simulink model "temp8"  (Simulink 7.7)
settings: Solver=ode45  SolverMode=SingleTasking  StartTime=0.0  StopTime=50  RelTol=1e-3
PreLoadFcn:
  | RefSignals
model workspace (MATLAB code in the model file):
  | commdvbt_tablegen
values from neighbouring files (symbols this model uses):
  Tsample = 9e3    (= 9000)    [RefSignals.m]
  VAR = {}    [RefSignals.m]
undefined symbols (not defined in the file or in its folder): Fs, get, rsgenpoly, sided, Two
libraries: dspmtrx3 x16, simulink x9, commblkintrlv2 x3, commutil2 x3, commblkcod2 x1, commcnvcod2 x1, commdigbbndam3 x1, dspxfrm3 x1, dspsnks4 x1, dspsigops x1, commcnvintrlv2 x1, commsdrhw_v2 x1
Description:
  | Digital Video Broadcasting - Terrestrial
CloseFcn:
  | % Clear global variables
  | clear global GF_TABLE1 GF_TABLE2 GF_TABLE_M GF_TABLE_PRIM_POLY
  | 
  | % Clear signal logging variable
  | clear dvbSigsOut
settings Model: Creator=The MathWorks Inc.  LastModifiedBy=katsikas  ExtModeTrigMode=oneshot  ExtModeArmWhenConnect=off  ExtModeAutoUpdateStatusClock=off  BufferReuse=off
settings SolverCC: ZeroCrossControl=DisableAll
settings DataIOCC: LimitDataPoints=off  SaveOutput=off  SaveTime=off  SignalLoggingName=dvbSigsOut
settings OptimizationCC: BlockReduction=off  BooleanDataType=off  OptimizeBlockIOStorage=off  BufferReuse=off  ExpressionFolding=off  LocalBlockOutputs=off  InitFltsAndDblsToZero=on  EfficientMapNaN2IntZero=off  OptimizeModelRefInitCode=on  LifeSpan=1  BufferReusableBoundary=off
settings DebuggingCC: SaveWithParameterizedLinksMsg=none  CheckExecutionContextPreStartOutputMsg=on  CheckExecutionContextRuntimeOutputMsg=on  SignalResolutionControl=TryResolveAllWithWarning  SolverPrmCheckMsg=none  InheritedTsInSrcMsg=none  MultiTaskDSMMsg=warning  MultiTaskCondExecSysMsg=none  SigSpecEnsureSampleTimeMsg=none  BusObjectLabelMismatch=none  StrictBusMsg=None
settings HardwareCC: TargetBitPerLong=64  TargetBitPerPointer=64  TargetEndianess=LittleEndian  TargetWordSize=64  TargetHWDeviceType=MATLAB Host
settings ModelReferenceCC: UpdateModelReferenceTargets=IfOutOfDate
settings RTWCC: SystemTargetFile=ert.tlc  TemplateMakefile=ert_default_tmf  Description=Real-Time Workshop Embedded Coder (no auto configuration)  RetainRTWFile=on  ProcessScript=ert_make_rtw_hook  IncludeERTFirstTime=on
settings CodeAppCC: IgnoreCustomStorageClasses=off
settings ERTTargetCC: TargetFcnLib=ansi_tfl_tmw.mat  FunctionExecutionProfile=off  MultiwordLength=2048  GenerateSampleERTMain=on  MatFileLogging=on  InlinedParameterPlacement=NonHierarchical  ERTCustomFileTemplate=example_file_process.tlc  ConvertIfToSwitch=off

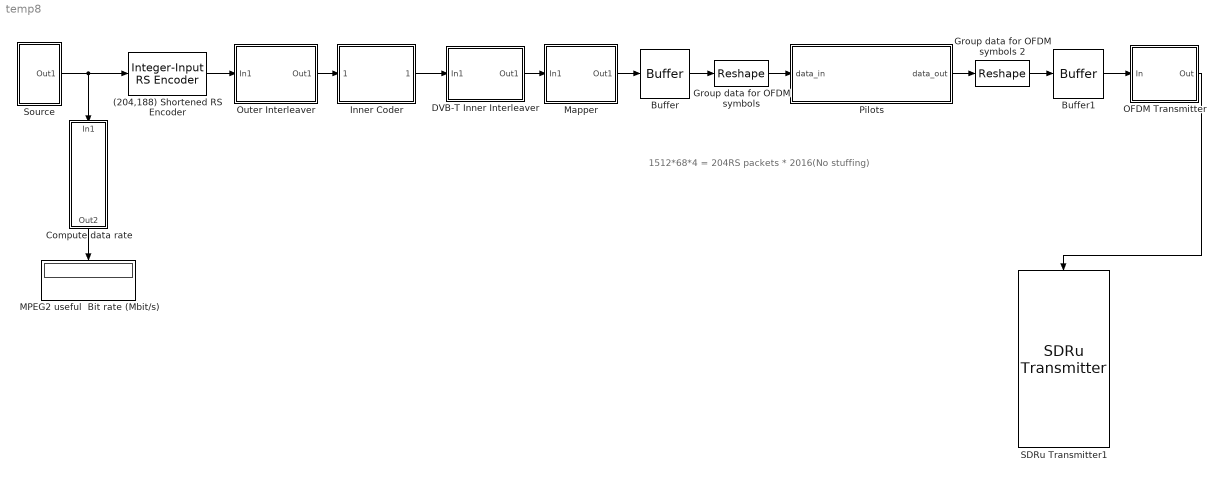
== system temp8 ==
  note: 1512*68*4 = 204RS packets * 2016(No stuffing)
  (204,188) Shortened RS Encoder : commblkcod2/Integer-Input RS Encoder  n=204  k=188  specPrimPoly=off  prPoly=[1 0 1 1]  specGenPoly=off  genPoly=rsgenpoly(7,3)  specPuncture=off  punctVec=[ones(2,1); zeros(2,1)]
  Buffer : Buffer  N=1512*68  TreatMby1Signals=One channel
  Buffer1 : Buffer  N=1705  TreatMby1Signals=One channel
  Compute data rate : Subsystem
      mask Display: disp(sprintf('Compute Bit\nRate (Mbit/s)'))
  DVB-T Inner Interleaver : Subsystem  mask(DVB-T Inner Interleaver){}
      mask init:
      | fullILVec = [(1:126) ...
      |  (rem([0:125]+63,126) +1 + 126     ) ...
      |  (rem([0:125]+105,126)+1 + (2*126) ) ...
      |  (rem([0:125]+42,126) +1 + (3*126) ) ...
      |  (rem([0:125]+21,126) +1 + (4*126) ) ...
      |  (rem([0:125]+84,126) +1 + (5*126) )];
      mask Display: disp('DVB-T\nInner\nInterleaver')
  "Group data for OFDM symbols " : Reshape  OutputDimensionality=Customize  OutputDimensions=[1512 68]
  Group data for OFDM symbols 2 : Reshape  OutputDimensionality=Column vector (2-D)  OutputDimensions=[1512 68]
  Inner Coder : Subsystem
      mask Display: disp('Rate 3/4\nPunctured\nConvolutional\nCode');
  MPEG2 useful  Bit rate (Mbit/s) : Display
      settings: Format=bank
  Mapper : Subsystem
      mask Type: DVB-T 64-QAM Mapper
      mask Display: disp('DVB-T\n64-QAM\nMapper')
  OFDM Transmitter : Subsystem
      mask Display: disp('OFDM\nTransmitter')
  Outer Interleaver : Subsystem
      mask Display: disp('Convolutional\nInterleaver\nI=12')
  Pilots : Stateflow chart  TreatAsAtomicUnit=on
  SDRu Transmitter1 : commsdrhw_v2/SDRu Transmitter  SystemSampleTime=-1  rxtx=tx  USRP2_IP='192.168.10.2'  centerFrequency=474e6  centerFrequencySrc=Dialog  loOffset=0  loOffsetSrc=Dialog  gain=20  gainSrc=Dialog  decimInterp=512  decimInterpSrc=Dialog  USRP2_IP_NUM=[49 57 50 46 49 54 56 46 49 48 46 50]  frameLength=362  outputDatatype=int16  overrunUnderrunPort=off  sampleTime=1  dboardInfo=|  HOST_DATA_PORT=30000  HOST_CONTROL_PORT=30001  USRP2_DATA_PORT=32769  USRP2_CONTROL_PORT=32768
      | dbid: 0
      |           dbName: 'no db found'
      |          freqMin: 0
      |          freqMax: 0
      |          gainMin: 0
      |          gainMax: 0
      |     gainStepSize: 0
  Source : Subsystem
  wires:
  Source/1(Out1) -> Compute data rate/1(In1), (204,188) Shortened RS Encoder/1
  (204,188) Shortened RS Encoder/1 -> Outer Interleaver/1(In1)
  Outer Interleaver/1(Out1) -> Inner Coder/1(Uncoded symbols)
  ? -> ?
  DVB-T Inner Interleaver/1(Out1) -> Mapper/1(In1)
  Inner Coder/1(Coded bits) -> DVB-T Inner Interleaver/1(In1)
  Mapper/1(Out1) -> Buffer/1
  Buffer/1 -> "Group data for OFDM symbols "/1
  "Group data for OFDM symbols "/1 -> Pilots/1(data_in)
  Pilots/1(data_out) -> Group data for OFDM symbols 2/1
  Compute data rate/1(Out2) -> MPEG2 useful  Bit rate (Mbit/s)/1
  OFDM Transmitter/1(Out) -> SDRu Transmitter1/1
  Buffer1/1 -> OFDM Transmitter/1(In)
  Group data for OFDM symbols 2/1 -> Buffer1/1

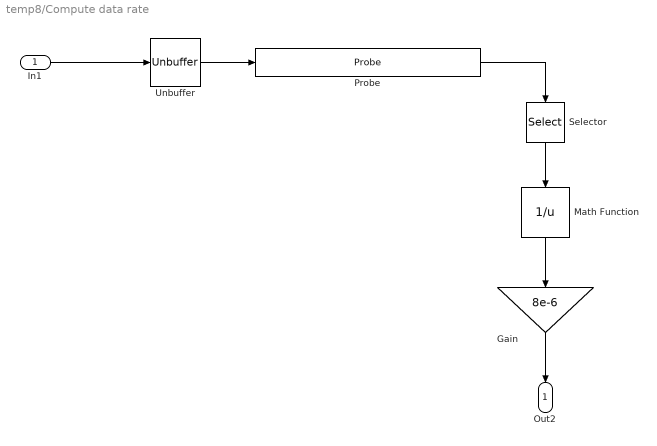
== system temp8/Compute data rate ==
  In1 : Inport
  Gain : Gain  Gain=8e-6
  Math Function : Math  Operator=reciprocal  SaturateOnIntegerOverflow=on
  Probe : Probe  ProbeWidth=off  ProbeComplexSignal=off
  Selector : Selector  InputPortWidth=2  IndexOptions=Index vector (dialog)  Indices=1  OutputSizes=1
  Unbuffer : Unbuffer  SampleBasedProcessing=Same as frame based
  Out2 : Outport
  wires:
  Probe/1 -> Selector/1
  In1/1 -> Unbuffer/1
  Selector/1 -> Math Function/1
  Math Function/1 -> Gain/1
  Gain/1 -> Out2/1
  Unbuffer/1 -> Probe/1

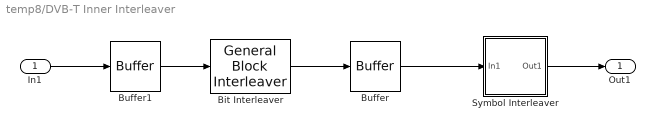
== system temp8/DVB-T Inner Interleaver ==
  In1 : Inport
  Bit Interleaver : commblkintrlv2/General Block Interleaver  elements=dvb_bit_int_table
  Buffer : Buffer  N=9072  TreatMby1Signals=One channel
  Buffer1 : Buffer  N=756  TreatMby1Signals=One channel
  Symbol Interleaver : Subsystem
      mask Display:
      | port_label('input', 1, '')
      | port_label('output', 1, '')
      | disp('Symbol\nInterleaver')
  Out1 : Outport
  wires:
  Buffer1/1 -> Bit Interleaver/1
  In1/1 -> Buffer1/1
  Bit Interleaver/1 -> Buffer/1
  Symbol Interleaver/1(Out1) -> Out1/1
  Buffer/1 -> Symbol Interleaver/1(In1)

== system temp8/Inner Coder ==
  Uncoded symbols : Inport
  Convolutional  Encoder : commcnvcod2/Convolutional Encoder  trellis=poly2trellis(7, [171 133])  opMode=Continuous  DelayedResetAction=off  hasIniStPort=off  hasFinStPort=off  usePuncVector=on  punctureVector=[1 1 0 1 1 0]'  reset=Unused parameter value
  Coded bits : Outport
  wires:
  Convolutional  Encoder/1 -> Coded bits/1
  Uncoded symbols/1 -> Convolutional  Encoder/1

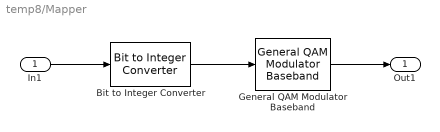
== system temp8/Mapper ==
  In1 : Inport
  Bit to Integer Converter : commutil2/Bit to Integer Converter  nbits=6  bitOrder=MSB first  signedOutputValues=Unsigned  outDtype=uint8  outDtypeSigned=Inherit via internal rule
  General QAM Modulator Baseband : commdigbbndam3/General QAM Modulator Baseband  SigCon=dvbt_qam  outDtype=double  outWordLen=16  outUDDataType=sfix(16)  outFracLenMode=Best precision  outFracLen=15
  Out1 : Outport
  wires:
  General QAM Modulator Baseband/1 -> Out1/1
  In1/1 -> Bit to Integer Converter/1
  Bit to Integer Converter/1 -> General QAM Modulator Baseband/1

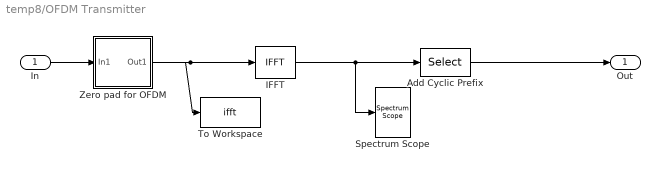
== system temp8/OFDM Transmitter ==
  In : Inport
  Add Cyclic Prefix : Selector  NumberOfDimensions=2  InputPortWidth=64  IndexOptions=Index vector (dialog),Select all  Indices=VAR.CyclicPrefixTX,-1  OutputSizes=1
  IFFT : dspxfrm3/IFFT  CompMethod=Table lookup  TableOpt=HYBRID  TableOptActive=Speed  BitRevOrder=off  cs_in=off  SkipNorm=on  InheritFFTLength=on  FFTLength=64  mode=Complex  outSamplingMode=Frame based  RowConvenienceOn=on  firstCoeffMode=User-defined  firstCoeffWordLength=16  firstCoeffFracLength=15  firstCoeffDataTypeStr=fixdt(1,16)  firstCoeffLastDataTypeStr=fixdt(1,16)  outputMin=[]  outputMax=[]  accumDataTypeStr=Inherit: Same as product output  accumLastDataTypeStr=Inherit: Same as product output  roundingMode=Floor  overflowMode=off
  Spectrum Scope : dspsnks4/Spectrum Scope  SystemSampleTime=-1  ScopeProperties=on  Domain=Frequency  HorizSpan=1  UseBuffer=off  BufferSize=128  Overlap=0  TreatMby1Signals=One channel  inpFftLenInherit=off  FFTlength=128  numAvg=2  DisplayProperties=off  AxisGrid=on  Memory=off  FrameNumber=on  AxisLegend=off  AxisZoom=off  OpenScopeAtSimStart=on  OpenScopeImmediately=off  FigPos=get(0,'defaultfigureposition')  AxisProperties=off  XUnits=Hertz  XRange=Two-sided ((-Fs/2...Fs/2])  XDisplay=0  InheritXIncr=on  XIncr=1.0  XLabel=Samples  XLimit=Auto  YUnits=dBW/Hertz  XMax=1  XMin=0  YLabel=Magnitude-squared, dB  LineProperties=off  wintypeSpecScope=Hann  RsSpecScope=50  betaSpecScope=5  winsampSpecScope=Periodic  XAxisParamsVer=6.9  isFrameUpgraded=on
      settings: YMin=-10  YMax=10
  To Workspace : ToWorkspace  VariableName=ifft  SampleTime=-1  SaveFormat=Array
  Zero pad for OFDM : Subsystem
      mask Display: disp('Zero pad\nfor OFDM');
  Out : Outport
  wires:
  IFFT/1 -> Add Cyclic Prefix/1, Spectrum Scope/1
  In/1 -> Zero pad for OFDM/1(In1)
  Zero pad for OFDM/1(Out1) -> IFFT/1, To Workspace/1
  Add Cyclic Prefix/1 -> Out/1

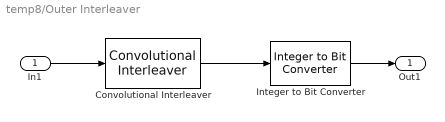
== system temp8/Outer Interleaver ==
  In1 : Inport
  Convolutional Interleaver : commcnvintrlv2/Convolutional Interleaver  SystemSampleTime=-1  N=12  B=17  ic=0
  Integer to Bit Converter : commutil2/Integer to Bit Converter  nbits=8  signedInputValues=Unsigned  bitOrder=MSB first  outDtype=boolean
  Out1 : Outport
  wires:
  Integer to Bit Converter/1 -> Out1/1
  Convolutional Interleaver/1 -> Integer to Bit Converter/1
  In1/1 -> Convolutional Interleaver/1

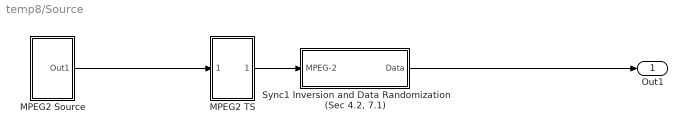
== system temp8/Source ==
  MPEG2 Source : Subsystem
  MPEG2 TS : Subsystem
  "Sync1 Inversion and Data Randomization (Sec 4.2, 7.1)" : Subsystem
  Out1 : Outport
  wires:
  MPEG2 Source/1(Out1) -> MPEG2 TS/1(In1)
  MPEG2 TS/1(MPEG-2 Trnsp) -> "Sync1 Inversion and Data Randomization (Sec 4.2, 7.1)"/1(MPEG-2)
  "Sync1 Inversion and Data Randomization (Sec 4.2, 7.1)"/1(Data) -> Out1/1

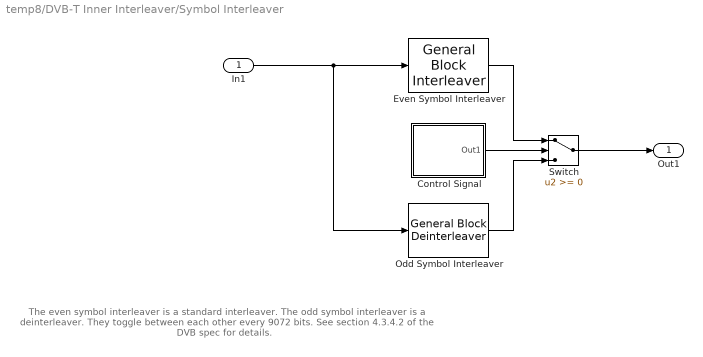
== system temp8/DVB-T Inner Interleaver/Symbol Interleaver ==
  note: The even symbol interleaver is a standard interleaver.  The odd symbol interleaver is a deinterleaver.  They toggle
      | between each other every 9072 bits.  See section 4.3.4.2 of the DVB spec for details.
  In1 : Inport
  Control Signal : Subsystem
      mask Display:
      | port_label('output', 1, 'ctrl')
      | disp('Control\nSignal')
  Even Symbol Interleaver : commblkintrlv2/General Block Interleaver  elements=dvb_sym_int_table
  Odd Symbol Interleaver : commblkintrlv2/General Block Deinterleaver  elements=dvb_sym_int_table
  Switch : Switch
  Out1 : Outport
  wires:
  In1/1 -> Even Symbol Interleaver/1, Odd Symbol Interleaver/1
  Switch/1 -> Out1/1
  Control Signal/1(Out1) -> Switch/2
  Even Symbol Interleaver/1 -> Switch/1
  Odd Symbol Interleaver/1 -> Switch/3

== system temp8/OFDM Transmitter/Zero pad for OFDM ==
  In1 : Inport
  Selector : Selector  NumberOfDimensions=2  InputPortWidth=2048  IndexOptions=Index vector (dialog),Select all  Indices="[1:852 1706:2048  853:1705],1"  OutputSizes=1,1
  Zero Pad : dspsigops/Pad  padAlong=Columns  dimsToPad=1  valSrc=Specify via dialog  padVal=0  spec=Output size  padNumOutRowsSpecMethod=User-specified  numOutRows=2048  padNumOutColsSpecMethod=User-specified  numOutCols=1  isVarDimsMode=off  padBeginning=0  padEnd=0  outSizeMode=User-specified  outSize=1  padSigAt=End  trunc_flag=None  roundingMode=Floor  overflowMode=off  truncOrWrapMode=Truncate  wrap_flag=None
  Out1 : Outport
  wires:
  In1/1 -> Zero Pad/1
  Selector/1 -> Out1/1
  Zero Pad/1 -> Selector/1

== system temp8/Source/MPEG2 Source ==
  Buffer : Buffer  N=184  TreatMby1Signals=One channel
  Read Binary File : vipsrcs/Read Binary File  FileName=/home/katsikas/katsikas-repo/Simulink/Korgialas_GeiaSou.ts  loopOrNot=on  numLoops=1  VideoFormat=Custom  FOURCC=I420  BitStreamFormat=Planar  NumOutputs=1  ComponentOrder=[1]  Interlaced=off  LineOrdering=Top line first  Ts=1/Tsample  Component1=Y'  Component2=Cb  Component3=Cr  Component4=Alpha  Bits1=8  Bits2=8  Bits3=8  Bits4=8  Rows1=512  Rows2=60  Rows3=60  Rows4=288  Cols1=736  Cols2=80  Cols3=80  Cols4=352  YRows=288  YCols=352  SignedOutput=off  FileEndian=Little endian  OutputEOF=off
  Reshape : Reshape  OutputDimensionality=Column vector (2-D)
  Out1 : Outport
  wires:
  Read Binary File/1 -> Reshape/1
  Reshape/1 -> Buffer/1
  Buffer/1 -> Out1/1

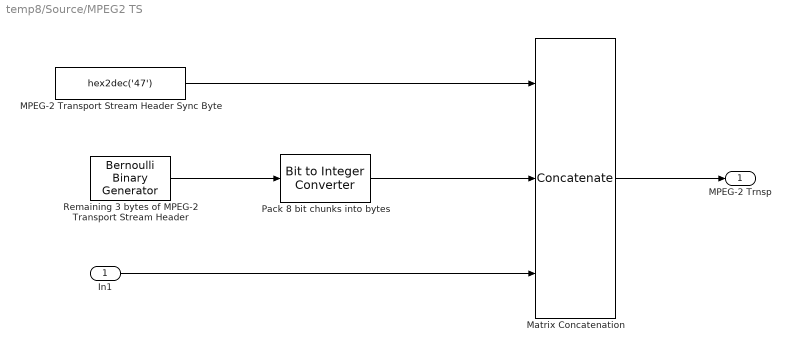
== system temp8/Source/MPEG2 TS ==
  In1 : Inport
  MPEG-2 Transport Stream Header Sync Byte : Constant  Value=hex2dec('47')  VectorParams1D=off  OutDataTypeStr=uint8  FramePeriod=8*188/Tsample
      settings: SamplingMode=Frame based
  Matrix Concatenation : Concatenate  NumInputs=3  Mode=Multidimensional array
  Pack 8 bit chunks into bytes : commutil2/Bit to Integer Converter  nbits=8  bitOrder=MSB first  signedOutputValues=Unsigned  outDtype=uint8  outDtypeSigned=Inherit via internal rule
  Remaining 3 bytes of MPEG-2 Transport Stream Header : commrandsrc2/Bernoulli Binary Generator  SystemSampleTime=-1  P=1  seed=61  Ts=(8*188/Tsample) / (3*8)  frameBased=on  sampPerFrame=3*8  orient=off  outDataType=uint8
  MPEG-2 Trnsp : Outport
  wires:
  MPEG-2 Transport Stream Header Sync Byte/1 -> Matrix Concatenation/1
  Remaining 3 bytes of MPEG-2 Transport Stream Header/1 -> Pack 8 bit chunks into bytes/1
  Matrix Concatenation/1 -> MPEG-2 Trnsp/1
  Pack 8 bit chunks into bytes/1 -> Matrix Concatenation/2
  In1/1 -> Matrix Concatenation/3

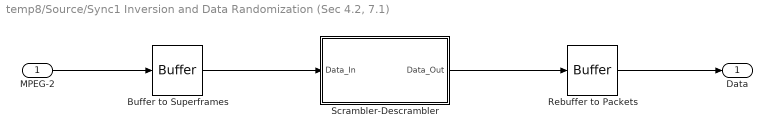
== system temp8/Source/Sync1 Inversion and Data Randomization (Sec 4.2, 7.1) ==
  MPEG-2 : Inport
  Buffer to Superframes : Buffer  N=1504  TreatMby1Signals=One channel
  Rebuffer to Packets : Buffer  N=188  TreatMby1Signals=One channel
  Scrambler-Descrambler : Subsystem
  Data : Outport
  wires:
  MPEG-2/1 -> Buffer to Superframes/1
  Rebuffer to Packets/1 -> Data/1
  Buffer to Superframes/1 -> Scrambler-Descrambler/1(Data_In)
  Scrambler-Descrambler/1(Data_Out) -> Rebuffer to Packets/1

== system temp8/DVB-T Inner Interleaver/Symbol Interleaver/Control Signal ==
  note: Generate a control signal that toggles between +/- 1 every frame of 9072 bits
  DSP Constant1 : Constant  VectorParams1D=off
  Pulse Generator : DiscretePulseGenerator  Amplitude=2  SampleTime=-1
  Subtract : Sum  Inputs=|+-
  Out1 : Outport
  wires:
  Subtract/1 -> Out1/1
  DSP Constant1/1 -> Subtract/2
  Pulse Generator/1 -> Subtract/1

== system temp8/Source/Sync1 Inversion and Data Randomization (Sec 4.2, 7.1)/Scrambler-Descrambler ==
  Data_In : Inport
  PRBS : Subsystem
  XOR and Concatenate : Subsystem
  Data_Out : Outport
  wires:
  PRBS/1(PRBS1) -> XOR and Concatenate/2(PRBS1)
  PRBS/2(PRBS2) -> XOR and Concatenate/3(PRBS2)
  PRBS/3(PRBS3) -> XOR and Concatenate/4(PRBS3)
  PRBS/4(PRBS4) -> XOR and Concatenate/5(PRBS4)
  PRBS/5(PRBS5) -> XOR and Concatenate/6(PRBS5)
  PRBS/6(PRBS6) -> XOR and Concatenate/7(PRBS6)
  PRBS/7(PRBS7) -> XOR and Concatenate/8(PRBS7)
  PRBS/8(PRBS8) -> XOR and Concatenate/9(PRBS8)
  Data_In/1 -> XOR and Concatenate/1(Data)
  XOR and Concatenate/1(Out1) -> Data_Out/1

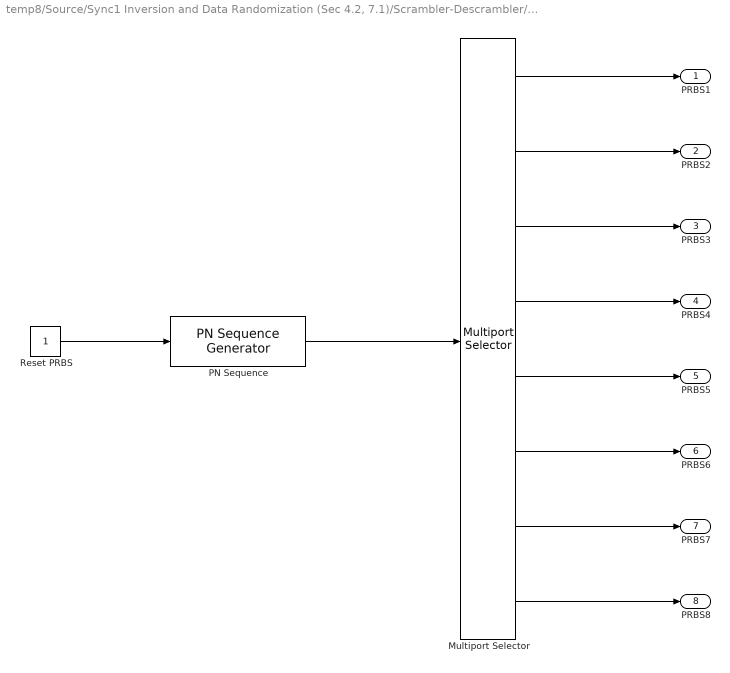
== system temp8/Source/Sync1 Inversion and Data Randomization (Sec 4.2, 7.1)/Scrambler-Descrambler/PRBS ==
  Multiport Selector : dspindex/Multiport Selector  rowsOrCols=Rows  idxCellArray={[1:187], [189:375], [377:563], [565:751], [753:939], [941:1127], [1129:1315], [1317:1503]}  idxErrMode=Clip Index
  PN Sequence : commseqgen2/PN Sequence Generator  poly=[15 14 0]  ini_sta=[1 0 0 1 0 1 0 1 0 0 0 0 0 0 0]  outBitMaskSource=Dialog parameter  shift=15  outVarSiz=off  maxOutSizeMode=Dialog parameter  maxOutSize=[10 1]  Ts=8 * (8*188/Tsample) / (8*188 - 1)  frameBased=on  sampPerFrame=(8*188 - 1)  reset=on  bitPackedOutputs=on  outDataType=Smallest unsigned integer  numPackedBits=8  bitPackDataSigned=off  bitPackedOutDType=Smallest integer
  Reset PRBS : Constant  VectorParams1D=off  OutDataTypeStr=boolean  SampleTime=8 * (8*188/Tsample)
  PRBS1 : Outport
  PRBS2 : Outport  Port=2
  PRBS3 : Outport  Port=3
  PRBS4 : Outport  Port=4
  PRBS5 : Outport  Port=5
  PRBS6 : Outport  Port=6
  PRBS7 : Outport  Port=7
  PRBS8 : Outport  Port=8
  wires:
  PN Sequence/1 -> Multiport Selector/1
  Multiport Selector/1 -> PRBS1/1
  Multiport Selector/2 -> PRBS2/1
  Multiport Selector/3 -> PRBS3/1
  Multiport Selector/4 -> PRBS4/1
  Multiport Selector/5 -> PRBS5/1
  Multiport Selector/6 -> PRBS6/1
  Multiport Selector/7 -> PRBS7/1
  Multiport Selector/8 -> PRBS8/1
  Reset PRBS/1 -> PN Sequence/1

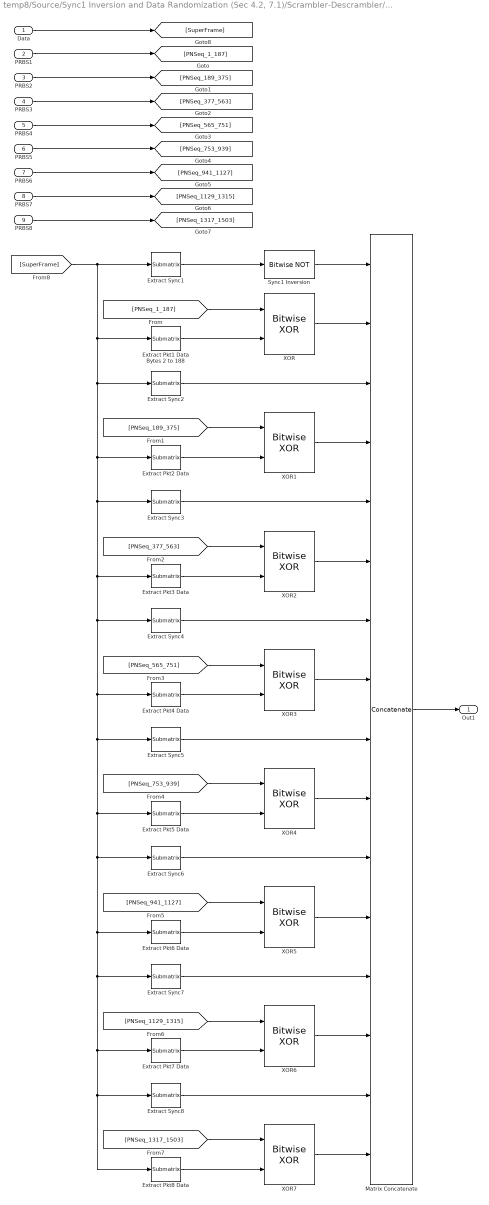
== system temp8/Source/Sync1 Inversion and Data Randomization (Sec 4.2, 7.1)/Scrambler-Descrambler/XOR and Concatenate ==
  Data : Inport
  PRBS1 : Inport  Port=2
  PRBS2 : Inport  Port=3
  PRBS3 : Inport  Port=4
  PRBS4 : Inport  Port=5
  PRBS5 : Inport  Port=6
  PRBS6 : Inport  Port=7
  PRBS7 : Inport  Port=8
  PRBS8 : Inport  Port=9
  Extract Pkt1 Data Bytes 2 to 188 : dspmtrx3/Submatrix  RowSpan=Range of rows  RowStartMode=Index  RowStartIndex=2  RowEndMode=Index  RowEndIndex=188  ColSpan=All columns  ColStartMode=First  ColStartIndex=1  ColEndMode=Last  ColEndIndex=1
  Extract Pkt2 Data : dspmtrx3/Submatrix  RowSpan=Range of rows  RowStartMode=Index  RowStartIndex=188+2  RowEndMode=Index  RowEndIndex=2*188  ColSpan=All columns  ColStartMode=First  ColStartIndex=1  ColEndMode=Last  ColEndIndex=1
  Extract Pkt3 Data : dspmtrx3/Submatrix  RowSpan=Range of rows  RowStartMode=Index  RowStartIndex=2*188+2  RowEndMode=Index  RowEndIndex=3*188  ColSpan=All columns  ColStartMode=First  ColStartIndex=1  ColEndMode=Last  ColEndIndex=1
  Extract Pkt4 Data : dspmtrx3/Submatrix  RowSpan=Range of rows  RowStartMode=Index  RowStartIndex=3*188+2  RowEndMode=Index  RowEndIndex=4*188  ColSpan=All columns  ColStartMode=First  ColStartIndex=1  ColEndMode=Last  ColEndIndex=1
  Extract Pkt5 Data : dspmtrx3/Submatrix  RowSpan=Range of rows  RowStartMode=Index  RowStartIndex=4*188+2  RowEndMode=Index  RowEndIndex=5*188  ColSpan=All columns  ColStartMode=First  ColStartIndex=1  ColEndMode=Last  ColEndIndex=1
  Extract Pkt6 Data : dspmtrx3/Submatrix  RowSpan=Range of rows  RowStartMode=Index  RowStartIndex=5*188+2  RowEndMode=Index  RowEndIndex=6*188  ColSpan=All columns  ColStartMode=First  ColStartIndex=1  ColEndMode=Last  ColEndIndex=1
  Extract Pkt7 Data : dspmtrx3/Submatrix  RowSpan=Range of rows  RowStartMode=Index  RowStartIndex=6*188+2  RowEndMode=Index  RowEndIndex=7*188  ColSpan=All columns  ColStartMode=First  ColStartIndex=1  ColEndMode=Last  ColEndIndex=1
  Extract Pkt8 Data : dspmtrx3/Submatrix  RowSpan=Range of rows  RowStartMode=Index  RowStartIndex=7*188+2  RowEndMode=Last  RowEndIndex=8*188  ColSpan=All columns  ColStartMode=First  ColStartIndex=1  ColEndMode=Last  ColEndIndex=1
  Extract Sync1 : dspmtrx3/Submatrix  RowSpan=One row  RowStartMode=First  RowStartIndex=1  RowEndMode=Index  RowEndIndex=8  ColSpan=All columns  ColStartMode=First  ColStartIndex=1  ColEndMode=Last  ColEndIndex=1
  Extract Sync2 : dspmtrx3/Submatrix  RowSpan=One row  RowStartMode=Index  RowStartIndex=188+1  RowEndMode=Index  RowEndIndex=8  ColSpan=All columns  ColStartMode=First  ColStartIndex=1  ColEndMode=Last  ColEndIndex=1
  Extract Sync3 : dspmtrx3/Submatrix  RowSpan=One row  RowStartMode=Index  RowStartIndex=2*188+1  RowEndMode=Index  RowEndIndex=8  ColSpan=All columns  ColStartMode=First  ColStartIndex=1  ColEndMode=Last  ColEndIndex=1
  Extract Sync4 : dspmtrx3/Submatrix  RowSpan=One row  RowStartMode=Index  RowStartIndex=3*188+1  RowEndMode=Index  RowEndIndex=8  ColSpan=All columns  ColStartMode=First  ColStartIndex=1  ColEndMode=Last  ColEndIndex=1
  Extract Sync5 : dspmtrx3/Submatrix  RowSpan=One row  RowStartMode=Index  RowStartIndex=4*188+1  RowEndMode=Index  RowEndIndex=8  ColSpan=All columns  ColStartMode=First  ColStartIndex=1  ColEndMode=Last  ColEndIndex=1
  Extract Sync6 : dspmtrx3/Submatrix  RowSpan=One row  RowStartMode=Index  RowStartIndex=5*188+1  RowEndMode=Index  RowEndIndex=8  ColSpan=All columns  ColStartMode=First  ColStartIndex=1  ColEndMode=Last  ColEndIndex=1
  Extract Sync7 : dspmtrx3/Submatrix  RowSpan=One row  RowStartMode=Index  RowStartIndex=6*188+1  RowEndMode=Index  RowEndIndex=8  ColSpan=All columns  ColStartMode=First  ColStartIndex=1  ColEndMode=Last  ColEndIndex=1
  Extract Sync8 : dspmtrx3/Submatrix  RowSpan=One row  RowStartMode=Index  RowStartIndex=7*188+1  RowEndMode=Index  RowEndIndex=8  ColSpan=All columns  ColStartMode=First  ColStartIndex=1  ColEndMode=Last  ColEndIndex=1
  Matrix Concatenate : Concatenate  NumInputs=16  Mode=Multidimensional array
  Sync1 Inversion : simulink/Logic and Bit Operations/Bitwise Operator  logicop=NOT  UseBitMask=off  BitMask=bin2dec('11011001')  BitMaskRealWorld=Stored Integer
  XOR{,1..7} (8 alike) : simulink/Logic and Bit Operations/Bitwise Operator  logicop=XOR  UseBitMask=off  NumInputPorts=2  BitMask=bin2dec('11011001')  BitMaskRealWorld=Stored Integer
  Out1 : Outport
  wires:
  [SuperFrame] -> Extract Pkt2 Data/1, Extract Pkt3 Data/1, Extract Pkt4 Data/1, Extract Pkt5 Data/1, Extract Pkt6 Data/1, Extract Pkt8 Data/1, Extract Sync8/1, Extract Pkt7 Data/1, Extract Sync7/1, Extract Sync6/1, Extract Sync5/1, Extract Sync4/1, Extract Sync3/1, Extract Sync2/1, Extract Pkt1 Data Bytes 2 to 188/1, Extract Sync1/1
  Extract Sync1/1 -> Sync1 Inversion/1
  Extract Pkt1 Data Bytes 2 to 188/1 -> XOR/2
  [PNSeq_1_187] -> XOR/1
  Sync1 Inversion/1 -> Matrix Concatenate/1
  XOR/1 -> Matrix Concatenate/2
  Extract Sync2/1 -> Matrix Concatenate/3
  Extract Sync3/1 -> Matrix Concatenate/5
  Extract Sync4/1 -> Matrix Concatenate/7
  Extract Sync5/1 -> Matrix Concatenate/9
  Extract Sync6/1 -> Matrix Concatenate/11
  Extract Sync7/1 -> Matrix Concatenate/13
  Extract Sync8/1 -> Matrix Concatenate/15
  XOR1/1 -> Matrix Concatenate/4
  XOR2/1 -> Matrix Concatenate/6
  XOR3/1 -> Matrix Concatenate/8
  XOR4/1 -> Matrix Concatenate/10
  XOR5/1 -> Matrix Concatenate/12
  XOR6/1 -> Matrix Concatenate/14
  XOR7/1 -> Matrix Concatenate/16
  [PNSeq_189_375] -> XOR1/1
  [PNSeq_377_563] -> XOR2/1
  [PNSeq_565_751] -> XOR3/1
  [PNSeq_753_939] -> XOR4/1
  [PNSeq_941_1127] -> XOR5/1
  [PNSeq_1129_1315] -> XOR6/1
  [PNSeq_1317_1503] -> XOR7/1
  Extract Pkt2 Data/1 -> XOR1/2
  Extract Pkt3 Data/1 -> XOR2/2
  Extract Pkt4 Data/1 -> XOR3/2
  Extract Pkt5 Data/1 -> XOR4/2
  Extract Pkt6 Data/1 -> XOR5/2
  Extract Pkt7 Data/1 -> XOR6/2
  Extract Pkt8 Data/1 -> XOR7/2
  Matrix Concatenate/1 -> Out1/1
  PRBS1/1 -> [PNSeq_1_187]
  PRBS2/1 -> [PNSeq_189_375]
  PRBS3/1 -> [PNSeq_377_563]
  PRBS4/1 -> [PNSeq_565_751]
  PRBS5/1 -> [PNSeq_753_939]
  PRBS6/1 -> [PNSeq_941_1127]
  PRBS7/1 -> [PNSeq_1129_1315]
  PRBS8/1 -> [PNSeq_1317_1503]
  Data/1 -> [SuperFrame]

== matlab function Pilots ==
  data: data_in input double; data_out output double; VAR parameter double
function data_out = insert_reference_signals(data_in, VAR)
  
  w = VAR.w;
  symbols = 68;
  used_carriers = 1705;
  tps_set = VAR.tps_signals;
  pilot_set = VAR.pilot_set;
  

  % merge data and pilots
  temp = zeros(1705,68);
  data_out = complex(temp,0);
  for l=1:symbols
    v = 1; % current input payload carrier index
    pilot = 1; % current pilot index in pilot_set
    tps=1; % current tps index in tps_set
        for u = 1:used_carriers % for all output carriers
            p = 1+pilot_set(pilot); % get next pilot
            if tps <= length(tps_set) % get next tps
                t = 1+tps_set(tps); 
            else
                t = 0;
            end

            if u == p % it's a pilot signal
                real = 4/3 * 2 * (0.5 - w(p));
                data_out(u,l) = complex(real);
                pilot = pilot + 1;
            elseif u == t; % it's a TPS signal
                real = 2 * (0.5 - w(p));
                %% comm.DBPSKModulator(pi/4);
                data_out(u,l) = complex(real);
                tps = tps + 1;
            else % it's a payload carrier
                data_out(u,l) = data_in(v);
                v = v + 1;
            end
        end
  end
  
  %data_out(:,1)
